simulink model "body_test"  (R2016b)
settings: Solver=FixedStepAuto  StartTime=0.0  StopTime=3200  FixedStep=Ts  RelTol=1e-3
values from neighbouring files (symbols this model uses):
  g = 9.80665    [Init_PI_reg.m]    (also in Initial_test.m; battery_test_res.mat; body_test_res.mat; motor_test_res.mat)
  k_drag = (1/2)*air_density*SCx    (= 0.435741)    [Init_PI_reg.m]    (also in Initial_test.m; battery_test_res.mat; body_test_res.mat; motor_test_res.mat)
  k_rolling = 0.013*m*g    (= 224.376152)    [Init_PI_reg.m]    (also in Initial_test.m; battery_test_res.mat; body_test_res.mat; motor_test_res.mat)
  m = 1600+80*2    (= 1760)    [Init_PI_reg.m]    (also in Initial_test.m; battery_test_res.mat; body_test_res.mat; motor_test_res.mat)
  mps_to_kmph = 3.6    [Init_PI_reg.m]    (also in Initial_test.m; battery_test_res.mat; body_test_res.mat; motor_test_res.mat)
  tourque_2_thrust = (2*pi*3.6/60)/rmp_2_kmph    (= 27.5392012014)    [Init_PI_reg.m]    (also in Initial_test.m; battery_test_res.mat; body_test_res.mat; motor_test_res.mat)
  Velocity_0 = 0    [Init_PI_reg.m]    (also in Initial_test.m; battery_test_res.mat; body_test_res.mat; motor_test_res.mat)
settings Model: Creator=a037702  LastModifiedBy=a037702

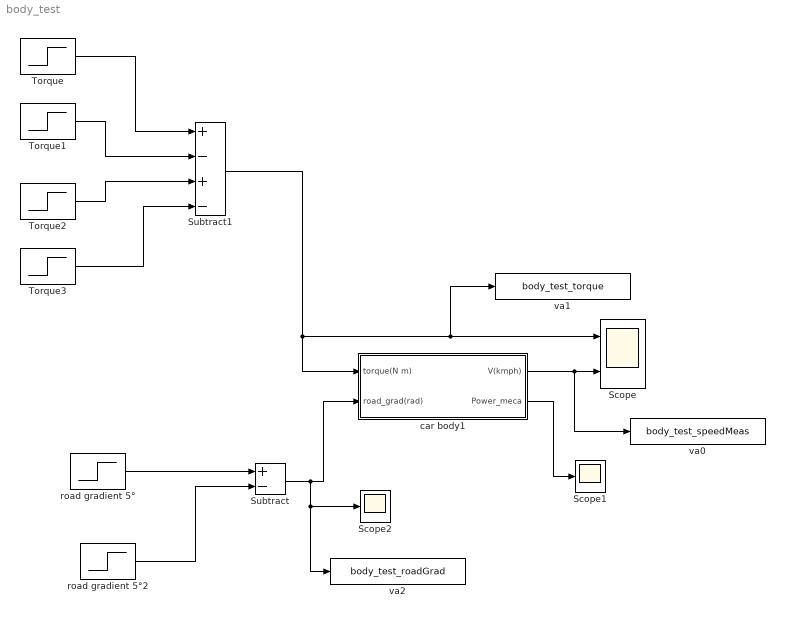
== system body_test ==
  Scope : Scope  NumInputPorts=2
  Scope1 : Scope
  Scope2 : Scope
  Subtract : Sum  Inputs=+-
  Subtract1 : Sum  Inputs=+-+-
  Torque : Step  Time=1400  Before=80  After=0  SampleTime=0
  Torque1 : Step  Time=2000  After=80  SampleTime=0
  Torque2 : Step  Time=2400  After=120  SampleTime=0
  Torque3 : Step  Time=2800  After=40  SampleTime=0
  car body1 : Subsystem
  road gradient 5° : Step  Time=500  After=5*(pi/180)  SampleTime=0
  road gradient 5°2 : Step  Time=100  After=5*(pi/180)  SampleTime=0
  va0 : ToWorkspace  VariableName=body_test_speedMeas  SaveFormat=Structure With Time  SampleTime=-1
      settings: Save2DSignal=2-D array (concatenate along first dimension)
  va1 : ToWorkspace  VariableName=body_test_torque  SaveFormat=Structure With Time  SampleTime=-1
      settings: Save2DSignal=2-D array (concatenate along first dimension)
  va2 : ToWorkspace  VariableName=body_test_roadGrad  SaveFormat=Structure With Time  SampleTime=-1
      settings: Save2DSignal=2-D array (concatenate along first dimension)
  wires:
  car body1/1(V(kmph)) -> va0/1, Scope/2
  car body1/2(Power_meca) -> Scope1/1
  road gradient 5°/1 -> Subtract/1
  road gradient 5°2/1 -> Subtract/2
  Subtract/1 -> va2/1, Scope2/1, car body1/2(road_grad(rad))
  Subtract1/1 -> va1/1, Scope/1, car body1/1(torque(N m))
  Torque/1 -> Subtract1/1
  Torque1/1 -> Subtract1/2
  Torque2/1 -> Subtract1/3
  Torque3/1 -> Subtract1/4

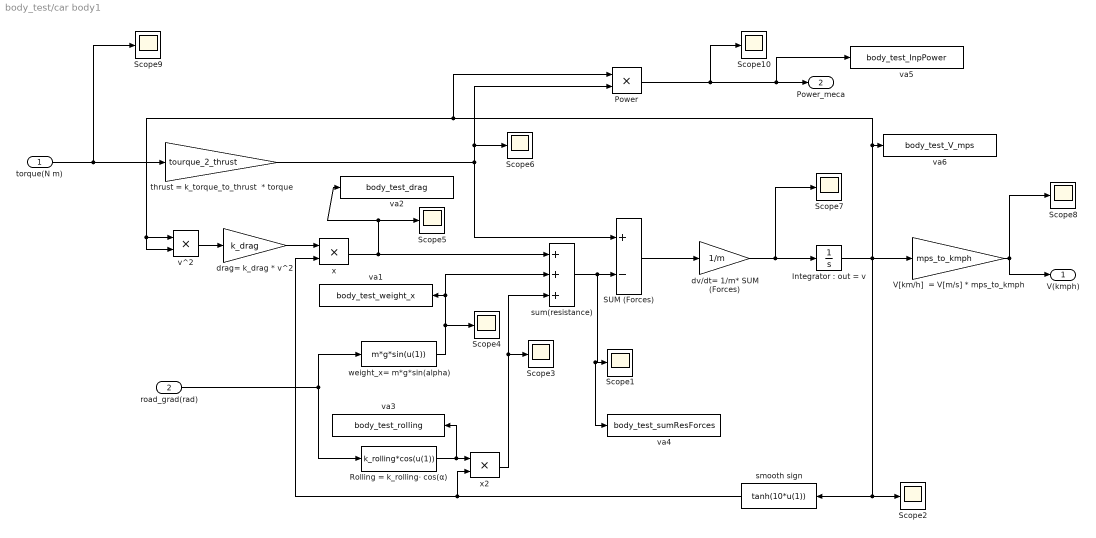
== system body_test/car body1 ==
  torque(N m) : Inport
  road_grad(rad) : Inport  Port=2
  "Integrator : out = v" : Integrator  InitialCondition=Velocity_0  LimitOutput=on  UpperSaturationLimit=400  LowerSaturationLimit=-400
  Power : Product
  Rolling = k_rolling· cos(α) : Fcn  Expr=k_rolling*cos(u(1))
  SUM (Forces) : Sum  Inputs=+-
  Scope{1..10} (10 alike) : Scope
  V[km/h]  = V[m/s] * mps_to_kmph : Gain  Gain=mps_to_kmph
  drag= k_drag * v^2 : Gain  Gain=k_drag
  dv/dt= 1/m* SUM (Forces) : Gain  Gain=1/m
  smooth sign : Fcn  Expr=tanh(10*u(1))
  sum(resistance) : Sum  Inputs=+++
  thrust = k_torque_to_thrust  * torque : Gain  Gain=tourque_2_thrust
  v^2 : Product
  va1 : ToWorkspace  VariableName=body_test_weight_x  SaveFormat=Structure With Time  SampleTime=-1
      settings: Save2DSignal=2-D array (concatenate along first dimension)
  va2 : ToWorkspace  VariableName=body_test_drag  SaveFormat=Structure With Time  SampleTime=-1
      settings: Save2DSignal=2-D array (concatenate along first dimension)
  va3 : ToWorkspace  VariableName=body_test_rolling  SaveFormat=Structure With Time  SampleTime=-1
      settings: Save2DSignal=2-D array (concatenate along first dimension)
  va4 : ToWorkspace  VariableName=body_test_sumResForces  SaveFormat=Structure With Time  SampleTime=-1
      settings: Save2DSignal=2-D array (concatenate along first dimension)
  va5 : ToWorkspace  VariableName=body_test_InpPower  SaveFormat=Structure With Time  SampleTime=-1
      settings: Save2DSignal=2-D array (concatenate along first dimension)
  va6 : ToWorkspace  VariableName=body_test_V_mps  SaveFormat=Structure With Time  SampleTime=-1
      settings: Save2DSignal=2-D array (concatenate along first dimension)
  weight_x= m*g*sin(alpha) : Fcn  Expr=m*g*sin(u(1))
  "x " : Product
  x2 : Product
  V(kmph) : Outport
  Power_meca : Outport  Port=2
  wires:
  weight_x= m*g*sin(alpha)/1 -> va1/1, sum(resistance)/2, Scope4/1
  thrust = k_torque_to_thrust  * torque/1 -> SUM (Forces)/1, Power/2, Scope6/1
  v^2/1 -> drag= k_drag * v^2/1
  V[km/h]  = V[m/s] * mps_to_kmph/1 -> V(kmph)/1, Scope8/1
  "Integrator : out = v"/1 -> Scope2/1, smooth sign/1, V[km/h]  = V[m/s] * mps_to_kmph/1, va6/1, Power/1, v^2/2, v^2/1
  dv/dt= 1/m* SUM (Forces)/1 -> "Integrator : out = v"/1, Scope7/1
  SUM (Forces)/1 -> dv/dt= 1/m* SUM (Forces)/1
  torque(N m)/1 -> Scope9/1, thrust = k_torque_to_thrust  * torque/1
  "x "/1 -> sum(resistance)/1, va2/1, Scope5/1
  road_grad(rad)/1 -> Rolling = k_rolling· cos(α)/1, weight_x= m*g*sin(alpha)/1
  Power/1 -> Scope10/1, va5/1, Power_meca/1
  Rolling = k_rolling· cos(α)/1 -> va3/1, x2/1
  x2/1 -> sum(resistance)/3, Scope3/1
  drag= k_drag * v^2/1 -> "x "/1
  smooth sign/1 -> "x "/2, x2/2
  sum(resistance)/1 -> va4/1, Scope1/1, SUM (Forces)/2
